simulink model "Key_harness"  (Simulink 7.7)
settings: Solver=FixedStepDiscrete  SolverMode=SingleTasking  StartTime=0.0  StopTime=100  FixedStep=0.01  RelTol=1e-3
PostLoadFcn:
  | load key.mat
undefined symbols (not defined in the file): ACTIVE, CD_KEY_DEBOUNCE_OFF, INACTIVE, MULTIPLE, sigbuilder_block, srate
CloseFcn:
  | rtwprivate ssgencode ModelCloseRequest sle_main_controller
settings Model: Creator=smindema  LastModifiedBy=aliebel  CovMetricSettings=dcmw  CovCumulativeReport=on
settings MATStruct: SampleTime=0.01  Offset=0  Priority=[1.0]
settings DataIOCC: LimitDataPoints=off  SaveOutput=off  SaveTime=off
settings OptimizationCC: BlockReduction=off  InlineParams=on  ExpressionFolding=off  StateBitsets=on  DataBitsets=on  UseTempVars=on  InitFltsAndDblsToZero=on  NoFixptDivByZeroProtection=on  EfficientFloat2IntCast=on  OptimizeModelRefInitCode=on
settings DebuggingCC: SaveWithParameterizedLinksMsg=none  MultiTaskDSMMsg=warning  MultiTaskCondExecSysMsg=none  IntegerOverflowMsg=none  ModelReferenceCSMismatchMessage=warning
settings HardwareCC: ProdBitPerInt=16  ProdBitPerPointer=16  ProdIntDivRoundTo=Floor  ProdEndianess=BigEndian  ProdWordSize=16  ProdHWDeviceType=Motorola HC12
settings ModelReferenceCC: ModelReferenceNumInstancesAllowed=Single
settings RTWCC: SystemTargetFile=ert.tlc  GenCodeOnly=on  TemplateMakefile=ert_default_tmf  Description=Real-Time Workshop Embedded Coder (no auto configuration)  GenerateReport=on  RetainRTWFile=on  ProcessScript=ert_make_rtw_hook  IncludeHyperlinkInReport=on  LaunchReport=on  IncludeERTFirstTime=on
settings RTWCC: CustomHeaderCode=|
  | #include "cpp_req_defines.h"
  | #include "hw_fin.h"
  | #include "cdata.h"
settings CodeAppCC: IgnoreCustomStorageClasses=off  DefineNamingRule=UpperCase
settings ERTTargetCC: TargetFcnLib=ansi_tfl_tmw.mat  FunctionExecutionProfile=off  MultiwordLength=2048  GenerateSampleERTMain=on  IncludeMdlTerminateFcn=off  SupportAbsoluteTime=off  SupportNonFinite=off  SupportComplex=off  PurelyIntegerCode=on  ERTCustomFileTemplate=gen_rtw_req_defines_h.tlc  GlobalDataDefinition=InSeparateSourceFile  GlobalDataReference=InSeparateHeaderFile  ConvertIfToSwitch=off

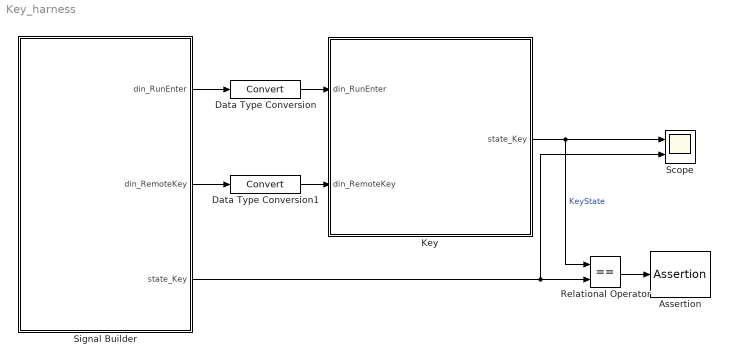
== system Key_harness ==
  Assertion : Assertion  Enabled=off
  Data Type Conversion : DataTypeConversion
  Data Type Conversion1 : DataTypeConversion
  Key : Subsystem  TreatAsAtomicUnit=on  SystemSampleTime=srate  RTWFileName=mod_Inputs
      settings: RTWSystemCode=Function  RTWFcnNameOpts=Use subsystem name  RTWFileNameOpts=User specified
  Relational Operator : RelationalOperator  Operator===  OutDataTypeStr=boolean
  Scope : Scope  NumInputPorts=2
      settings: YMin=-5~-5  YMax=5~5  MaxDataPoints=50000
  Signal Builder : Subsystem  Tag=STV Subsys  LoadFcn=sigbuilder_block('load');  StartFcn=sigbuilder_block('start');  StopFcn=sigbuilder_block('stop');  ClipboardFcn=sigbuilder_block('clipboard');  mask(Sigbuilder block){}
      mask help: Sigbuilder GUI
      mask init:
      | if ~strcmp(get_param(bdroot(gcbh),'SimulationStatus'),'stopped') tuvar = sigbuilder_block('maskInit'); end
      settings: CopyFcn=sigbuilder_block('copy');  DeleteFcn=sigbuilder_block('delete');  ModelCloseFcn=sigbuilder_block('modelClose');  PreSaveFcn=sigbuilder_block('preSave');  NameChangeFcn=sigbuilder_block('namechange');  OpenFcn=sigbuilder_block('open',[69 110.25 1200 714 ]);  CloseFcn=sigbuilder_block('close');
      mask Display: plot(0,0,100,100,[10,10,40,40,10],[80,20,20,80,80],[40,10],[50,50], [40,27,10],[65,72,56],[40,25,25,10],[28,28,43,43]);
  wires:
  Key/1(state_Key) -> Scope/1, Relational Operator/1  "KeyState"
  Signal Builder/1(din_RunEnter) -> Data Type Conversion/1
  Signal Builder/2(din_RemoteKey) -> Data Type Conversion1/1
  Data Type Conversion/1 -> Key/1(din_RunEnter)
  Data Type Conversion1/1 -> Key/2(din_RemoteKey)
  Relational Operator/1 -> Assertion/1
  Signal Builder/3(state_Key) -> Relational Operator/2, Scope/2

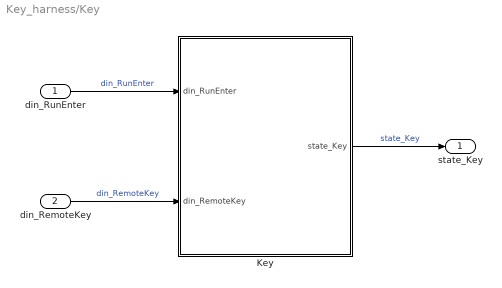
== system Key_harness/Key ==
  din_RunEnter : Inport
  din_RemoteKey : Inport  Port=2
  Key : Stateflow chart  TreatAsAtomicUnit=on
  state_Key : Outport
  wires:
  Key/1(state_Key) -> state_Key/1  "state_Key"
  din_RunEnter/1 -> Key/1(din_RunEnter)  "din_RunEnter"
  din_RemoteKey/1 -> Key/2(din_RemoteKey)  "din_RemoteKey"

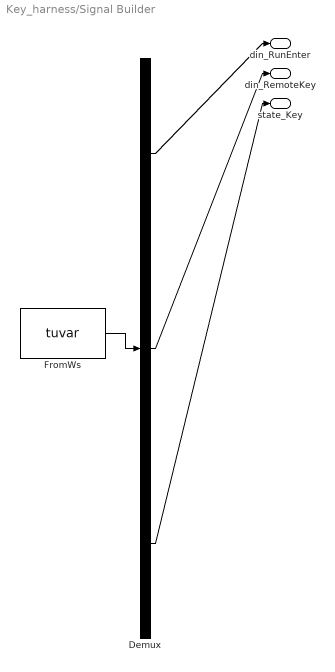
== system Key_harness/Signal Builder ==
  Demux : Demux  Tag=STV Demux  Outputs=3
  FromWs : FromWorkspace  Tag=STV FromWs  VariableName=tuvar  SampleTime=0  SigBuilderData=DataTag0  VnvData=DataTag1
      SigBuilderData=|
      | common.afterFinalStr = 'Extrapolate'
      | common.sampleTime = 0
      | dataSet(1).timeRange = [0 100]
      | dataSet(1).name = 'Group 2'
      | dataSet(2).timeRange = [0 100]
      | dataSet(2).name = 'Group 3'
      | sbobj.Groups(1).Name = 'Group 2'
      | sbobj.Groups(1).Signals(1).Name = 'din_RunEnter'
      | sbobj.Groups(1).Signals(1).XData = [0 7 7 15.8 15.8 35 35 42 42 49.6 49.6 64.8 64.8 73.2 73.2 87 87 100]
      | sbobj.Groups(1).Signals(1).YData = [0 0 1 1 0 0 1 1 0 0 1 1 0 0 1 1 0 0]
      | sbobj.Groups(1).Signals(2).Name = 'din_RemoteKey'
      | sbobj.Groups(1).Signals(2).XData = [0 11 11 25.4 25.4 35 35 42 42 52.8 52.8 57 57 62.6 62.6 74.8 74.8 100]
      | sbobj.Groups(1).Signals(2).YData = [0 0 1 1 0 0 1 1 0 0 1 1 0 0 1 1 0 0]
      | sbobj.Groups(1).Signals(3).Name = 'state_Key'
      | sbobj.Groups(1).Signals(3).XData = [0 7 7 11 11 25.51 25.51 35 35 35.01 35.01 42.11 42.11 49.6 49.6 52.8 52.8 87.11 87.11 100]
      | sbobj.Groups(1).Signals(3).YData = [0 0 1 1 48 48 0 0 1 1 48 48 0 0 1 1 48 48 0 0]
      | sbobj.Groups(2).Name = 'Group 3'
      | sbobj.Groups(2).Signals(1).Name = 'din_RunEnter'
      | sbobj.Groups(2).Signals(1).XData = [0 7 7 15.8 15.8 35 35 42 42 49.6 49.6 64.8 64.8 73.2 73.2 87 87 92.4 92.4 93.7 93.7 93.79 93.79 100]
      | sbobj.Groups(2).Signals(1).YData = [0 0 1 1 0 0 1 1 0 0 1 1 0 0 1 1 0 0 1 1 0 0 1 1]
      | sbobj.Groups(2).Signals(2).Name = 'din_RemoteKey'
      | sbobj.Groups(2).Signals(2).XData = [0 18 18 25.4 25.4 35 35 42 42 52.8 52.8 57 57 62.6 62.6 74.8 74.8 100]
      | sbobj.Groups(2).Signals(2).YData = [0 0 1 1 0 0 1 1 0 0 1 1 0 0 1 1 0 0]
      | sbobj.Groups(2).Signals(3).Name = 'state_Key'
      | sbobj.Groups(2).Signals(3).XData = [0 7 7 15.91 15.91 18 18 25.51 25.51 35 35 35.01 35.01 42.11 42.11 49.6 49.6 52.8 52.8 87.11 87.11 92.4 92.4 100]
      | sbobj.Groups(2).Signals(3).YData = [0 0 1 1 0 0 1 1 0 0 1 1 48 48 0 0 1 1 48 48 0 0 1 1]
  din_RunEnter : Outport  Tag=STV Outport
  din_RemoteKey : Outport  Tag=STV Outport  Port=2
  state_Key : Outport  Tag=STV Outport  Port=3
  wires:
  FromWs/1 -> Demux/1
  Demux/1 -> din_RunEnter/1
  Demux/2 -> din_RemoteKey/1
  Demux/3 -> state_Key/1

== stateflow chart Key/Key ==
  settings: executeAtInitialization=1
  state KEY_STATE [parallel]
    settings: executionOrder=1
    state MULTIPLE
      en:state_Key = MULTIPLE;
    state ON
      en:state_Key = ACTIVE;
    state OFF
      state DEBOUNCE
        en:debounceCount = 0;
        du:debounceCount++;
      state OFF
        en:state_Key = INACTIVE;
      note: Turn key off right away with deluxe command.  Button is debounced
          | in panel.
      (default) -> DEBOUNCE
      DEBOUNCE -> KEY_STATE.OFF.OFF : [(debounceCount >= CD_KEY_DEBOUNCE_OFF)...
          | || (state_Key == INACTIVE)]
    (default) -> KEY_STATE.OFF
    KEY_STATE.OFF -> ON : [(din_RunEnter == ACTIVE)...
        | || (din_RemoteKey == ACTIVE)]
    ON -> KEY_STATE.OFF [order 1] : [(din_RunEnter == INACTIVE)...
        | && (din_RemoteKey == INACTIVE)]
    ON -> MULTIPLE [order 2] : [(din_RunEnter == ACTIVE )...
        | && (din_RemoteKey == ACTIVE)]
    MULTIPLE -> KEY_STATE.OFF : [(din_RunEnter == INACTIVE)...
        | && (din_RemoteKey == INACTIVE)]
  data: din_RunEnter input uint8; din_RemoteKey input uint8; state_Key output uint8; INACTIVE parameter uint8 =0; ACTIVE parameter uint8 =1; MULTIPLE parameter uint8 =48; debounceCount local uint16; CD_KEY_DEBOUNCE_OFF parameter uint16
